simulink model "test1"  (R2023b)
settings: Solver=VariableStepAuto  StartTime=0.0  StopTime=40.0  RelTol=1e-3
settings Model: Creator=francescafornasier  LastModifiedBy=francescafornasier

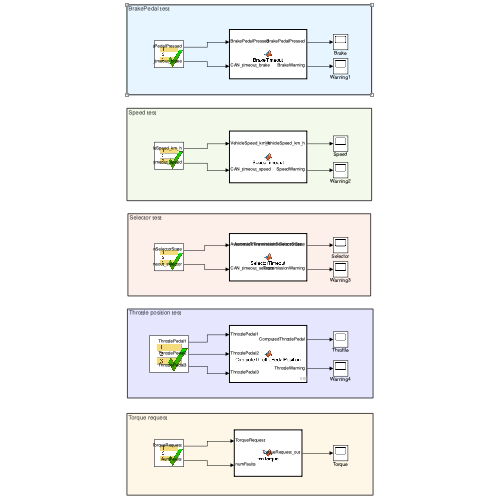
[thumbnail: Simulink's stored preview of the top-level diagram]
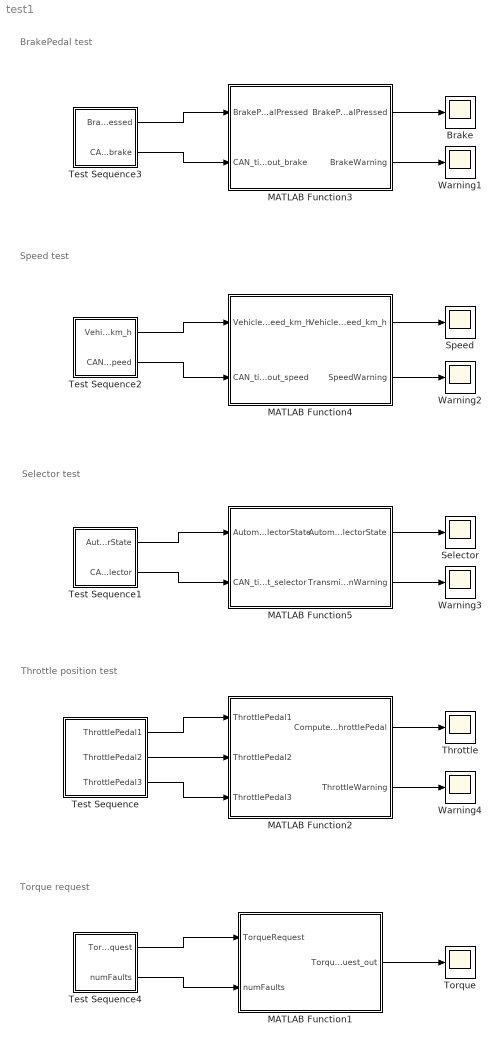
== system test1 ==
  note: Torque request
  note: Speed test
  note: Selector test
  note: Throttle position test
  note: BrakePedal test
  Brake : Scope
  MATLAB Function1 : MATLAB Function  TreatAsAtomicUnit=on
  MATLAB Function2 : MATLAB Function  TreatAsAtomicUnit=on
  MATLAB Function3 : MATLAB Function  TreatAsAtomicUnit=on
  MATLAB Function4 : MATLAB Function  TreatAsAtomicUnit=on
  MATLAB Function5 : MATLAB Function  TreatAsAtomicUnit=on
  Selector : Scope
  Speed : Scope
  Test Sequence : Test Sequence  TreatAsAtomicUnit=on
  Test Sequence1 : Test Sequence  TreatAsAtomicUnit=on
  Test Sequence2 : Test Sequence  TreatAsAtomicUnit=on
  Test Sequence3 : Test Sequence  TreatAsAtomicUnit=on
  Test Sequence4 : Test Sequence  TreatAsAtomicUnit=on
  Throttle : Scope
  Torque : Scope
  Warning{1..4} (4 alike) : Scope
  wires:
  Test Sequence/1(ThrottlePedal1) -> MATLAB Function2/1(ThrottlePedal1)
  Test Sequence/2(ThrottlePedal2) -> MATLAB Function2/2(ThrottlePedal2)
  Test Sequence/3(ThrottlePedal3) -> MATLAB Function2/3(ThrottlePedal3)
  MATLAB Function2/2(ThrottleWarning) -> Warning4/1
  MATLAB Function5/2(TransmissionWarning) -> Warning3/1
  MATLAB Function4/2(SpeedWarning) -> Warning2/1
  MATLAB Function3/2(BrakeWarning) -> Warning1/1
  MATLAB Function2/1(ComputedThrottlePedal) -> Throttle/1
  MATLAB Function5/1(AutomaticTransmissionSelectorState) -> Selector/1
  MATLAB Function3/1(BrakePedalPressed) -> Brake/1
  MATLAB Function4/1(VehicleSpeed_km_h) -> Speed/1
  Test Sequence2/2(CAN_timeout_speed) -> MATLAB Function4/2(CAN_timeout_speed)
  Test Sequence2/1(VehicleSpeed_km_h) -> MATLAB Function4/1("VehicleSpeed_km_h ")
  Test Sequence3/2(CAN_timeout_brake) -> MATLAB Function3/2(CAN_timeout_brake)
  Test Sequence3/1(BrakePedalPressed) -> MATLAB Function3/1("BrakePedalPressed ")
  Test Sequence1/1(AutomaticTransmissionSelectorState) -> MATLAB Function5/1("AutomaticTransmissionSelectorState ")
  Test Sequence1/2(CAN_timeout_selector) -> MATLAB Function5/2(CAN_timeout_selector)
  Test Sequence4/1(TorqueRequest) -> MATLAB Function1/1(TorqueRequest)
  Test Sequence4/2(numFaults) -> MATLAB Function1/2(numFaults)
  MATLAB Function1/1(TorqueRequest_out) -> Torque/1

== matlab function test1/MATLAB Function3 ==
  data: BrakePedalPressed input; CAN_timeout_brake input boolean; BrakePedalPressed output; BrakeWarning output single
function [BrakePedalPressed, BrakeWarning] = BrakeTimeout(BrakePedalPressed, CAN_timeout_brake)    
    if(CAN_timeout_brake==true)
        BrakePedalPressed=true;
        BrakeWarning=single(3);
    else
        BrakeWarning=single(0);
    end

== matlab function test1/MATLAB Function4 ==
  data: VehicleSpeed_km_h input; CAN_timeout_speed input boolean; VehicleSpeed_km_h output; SpeedWarning output single
function [VehicleSpeed_km_h, SpeedWarning]= SpeedTimeout(VehicleSpeed_km_h, CAN_timeout_speed)    
    if(CAN_timeout_speed==true)
        VehicleSpeed_km_h=single(0);
        SpeedWarning=single(4);
    else
        SpeedWarning=single(0);
    end

== matlab function test1/MATLAB Function5 ==
  data: AutomaticTransmissionSelectorState output; AutomaticTransmissionSelectorState input; CAN_timeout_selector input boolean; TransmissionWarning output single
function [AutomaticTransmissionSelectorState, TransmissionWarning] = SelectorTimeout(AutomaticTransmissionSelectorState, CAN_timeout_selector)    
    if(CAN_timeout_selector==true)
        TransmissionWarning = single(5);
    else
        TransmissionWarning = single(0);
    end

== stateflow chart test1/Test Sequence3 ==
  state step_1
    CAN_timeout_brake = true;
    BrakePedalPressed = true;
    settings: description=Data not up to date, BrakePedalPressed = true to allow driver to chande driving mode
  state step_2
    CAN_timeout_brake = false;
    BrakePedalPressed = true;
  state step_3
    CAN_timeout_brake = false;
    BrakePedalPressed = false;
  (default) -> step_1
  step_1 -> step_2 : [
      | after(5, sec)
      | ]
  step_2 -> step_3 : [
      | after(5, sec)
      | ]
  data: BrakePedalPressed output; CAN_timeout_brake output

== matlab function test1/MATLAB Function1 ==
  data: TorqueRequest input; numFaults input; TorqueRequest_out output
function TorqueRequest_out = fcnTorque(TorqueRequest, numFaults)
    if(numFaults==2)
        TorqueRequest_out = single(0);
    else
        TorqueRequest_out = TorqueRequest;
    end

== stateflow chart test1/Test Sequence4 ==
  state step_1
    numFaults = single(0);
    TorqueRequest = single(20);
  state step_2
    numFaults = single(1);
    TorqueRequest = single(30);
  state step_3
    numFaults = single(2);
    TorqueRequest = single(25);
  (default) -> step_1
  step_1 -> step_2 : [
      | after(5, sec)
      | ]
  step_2 -> step_3 : [
      | after(5, sec)
      | ]
  data: TorqueRequest output; numFaults output

== stateflow chart test1/Test Sequence1 ==
  state step_1
    CAN_timeout_selector = false;
    AutomaticTransmissionSelectorState = TransmissionState.Neutral;
  state step_2
    CAN_timeout_selector = true;
    AutomaticTransmissionSelectorState = TransmissionState.Drive;
  (default) -> step_1
  step_1 -> step_2 : [
      | after(5, sec)
      | ]
  data: AutomaticTransmissionSelectorState output Enum: TransmissionState; CAN_timeout_selector output

== matlab function test1/MATLAB Function2 ==
  data: ThrottlePedal1 input; ThrottlePedal2 input; ThrottlePedal3 input; ComputedThrottlePedal output single; ThrottleWarning output single
function [ComputedThrottlePedal,ThrottleWarning] = ComputeThrottlePedalPosition(ThrottlePedal1, ThrottlePedal2, ThrottlePedal3)
    tol = 0.05;
    ThrottleWarning=single(0);
    
    if(abs(ThrottlePedal1-ThrottlePedal2)<tol)
        if(abs(ThrottlePedal1-ThrottlePedal3)<tol && abs(ThrottlePedal2-ThrottlePedal3)<tol)
            ComputedThrottlePedal = mean([ThrottlePedal1 ThrottlePedal2 ThrottlePedal3]);
        else 
            ComputedThrottlePedal = mean([ThrottlePedal1 ThrottlePedal2]);
            ThrottleWarning = single(1);
        end
    elseif(abs(ThrottlePedal1-ThrottlePedal3)<tol)
            ComputedThrottlePedal = mean([ThrottlePedal1 ThrottlePedal3]);
            ThrottleWarning = single(1);
    elseif(abs(ThrottlePedal2-ThrottlePedal3)<tol)
            ComputedThrottlePedal = mean([ThrottlePedal2 ThrottlePedal3]);
            ThrottleWarning = single(1);
    else
        ThrottleWarning = single(2);
        ComputedThrottlePedal = single(-1);
    end

== stateflow chart test1/Test Sequence2 ==
  state step_1
    CAN_timeout_speed = false;
    VehicleSpeed_km_h = single(0);
  state step_2
    CAN_timeout_speed = true;
    VehicleSpeed_km_h = single(50);
  (default) -> step_1
  step_1 -> step_2 : [
      | after(5, sec)
      | ]
  data: VehicleSpeed_km_h output; CAN_timeout_speed output

== stateflow chart test1/Test Sequence ==
  state step_1
    ThrottlePedal1 = single(0.5);
    ThrottlePedal2 = single(0.52);
    ThrottlePedal3 =  single(0.51);
    settings: description=All 3 signals correct
  state step_2
    ThrottlePedal1 =  single(0.55);
    ThrottlePedal2 =  single(0.52);
    ThrottlePedal3 =  single(0.5);
    settings: description=Wrong signal 1
  state step_3
    ThrottlePedal1 =  single(0.5);
    ThrottlePedal2 =  single(0.55);
    ThrottlePedal3 =  single(0.52);
    settings: description=Wrong signal 2
  state step_4
    ThrottlePedal1 =  single(0.7);
    ThrottlePedal2 =  single(0.55);
    ThrottlePedal3 =  single(0.52);
    settings: description=Wrong signal 3
  state step_5
    ThrottlePedal1 =  single(0.5);
    ThrottlePedal2 =  single(0.55);
    ThrottlePedal3 =  single(0.45);
    settings: description=All signals are different
  state step_6
    ThrottlePedal1 =  single(0.8);
    ThrottlePedal2 =  single(0.72);
    ThrottlePedal3 =  single(0.74);
    settings: description=Wrong signal 1
  state step_7
    ThrottlePedal1 =  single(0.1);
    ThrottlePedal2 =  single(0.12);
    ThrottlePedal3 =  single(0.4);
    settings: description=Wrong signal 3
  (default) -> step_1
  step_1 -> step_2 : [
      | after(5, sec)
      | ]
  step_2 -> step_3 : [
      | after(5, sec)
      | ]
  step_3 -> step_4 : [
      | after(5, sec)
      | ]
  step_4 -> step_5 : [
      | after(5, sec)
      | ]
  step_5 -> step_6 : [
      | after(5, sec)
      | ]
  step_6 -> step_7 : [
      | after(5, sec)
      | ]
  data: ThrottlePedal1 output; ThrottlePedal2 output; ThrottlePedal3 output
